simulink library "GRC_Lib"  (R2017b)
settings: Solver=VariableStepAuto  StartTime=0.0  StopTime=10.0  RelTol=1e-3  EnableMultiTasking=on
StartFcn:
  | set_param('AdvancedOperations','ZoomFactor','100');
undefined symbols (not defined in the file): Test
libraries: GRC_Lib x203, simulink x1
(part 4 of 4)

== system GRC_Lib/ComparationOperation/aub ==
  Max : Inport
      settings: AttributesFormatString=%<OutDataTypeStr>
  u : Inport  Port=2
      settings: AttributesFormatString=%<OutDataTypeStr>
  Min : Inport  Port=3
      settings: AttributesFormatString=%<OutDataTypeStr>
  Logical Operator : Logic  AllPortsSameDT=off  OutDataTypeStr=boolean
  Relational Operator : RelationalOperator  OutDataTypeStr=boolean  RndMeth=Nearest
  Relational Operator1 : RelationalOperator  OutDataTypeStr=boolean  RndMeth=Nearest
  y : Outport
      settings: AttributesFormatString=%<OutDataTypeStr>
  wires:
  Relational Operator/1 -> Logical Operator/1
  Relational Operator1/1 -> Logical Operator/2
  Logical Operator/1 -> y/1
  u/1 -> Relational Operator1/1, Relational Operator/2
  Max/1 -> Relational Operator/1
  Min/1 -> Relational Operator1/2

== system GRC_Lib/ComparationOperation/uab ==
  Max : Inport
      settings: AttributesFormatString=%<OutDataTypeStr>
  u : Inport  Port=2
      settings: AttributesFormatString=%<OutDataTypeStr>
  Min : Inport  Port=3
      settings: AttributesFormatString=%<OutDataTypeStr>
  Logical Operator : Logic  AllPortsSameDT=off  OutDataTypeStr=boolean
  Relational Operator : RelationalOperator  OutDataTypeStr=boolean  RndMeth=Nearest
  Relational Operator1 : RelationalOperator  Operator=>  OutDataTypeStr=boolean  RndMeth=Nearest
  y : Outport
      settings: AttributesFormatString=%<OutDataTypeStr>
  wires:
  Relational Operator/1 -> Logical Operator/1
  Relational Operator1/1 -> Logical Operator/2
  Logical Operator/1 -> y/1
  u/1 -> Relational Operator1/1, Relational Operator/2
  Max/1 -> Relational Operator/1
  Min/1 -> Relational Operator1/2

== system GRC_Lib/ComparationOperation/uabu ==
  Max : Inport
      settings: AttributesFormatString=%<OutDataTypeStr>
  u : Inport  Port=2
      settings: AttributesFormatString=%<OutDataTypeStr>
  Min : Inport  Port=3
      settings: AttributesFormatString=%<OutDataTypeStr>
  Logical Operator : Logic  AllPortsSameDT=off  OutDataTypeStr=boolean
  Relational Operator : RelationalOperator  Operator=>  OutDataTypeStr=boolean  RndMeth=Nearest
  Relational Operator1 : RelationalOperator  Operator=>  OutDataTypeStr=boolean  RndMeth=Nearest
  y : Outport
      settings: AttributesFormatString=%<OutDataTypeStr>
  wires:
  Relational Operator/1 -> Logical Operator/1
  Relational Operator1/1 -> Logical Operator/2
  Logical Operator/1 -> y/1
  u/1 -> Relational Operator1/1, Relational Operator/2
  Max/1 -> Relational Operator/1
  Min/1 -> Relational Operator1/2

== system GRC_Lib/Constants_Parameters/CalConstant ==
  CalParam : Constant  Value=CalParamName
  Out : Outport
  wires:
  CalParam/1 -> Out/1

== system GRC_Lib/Constants_Parameters/Stdrd1DLookupTable ==
  u : Inport
      settings: AttributesFormatString=%<OutDataTypeStr>
  Stdrd1DTable : Lookup_n-D  NumberOfTableDimensions=1  BreakpointsForDimension1=[-pi:pi/50:pi]  BreakpointsForDimension1DataTypeStr=double  Table=sin([-pi:pi/50:pi])  TableDataTypeStr=double  IntermediateResultsDataTypeStr=double  InternalRulePriority=Speed  OutDataTypeStr=double  RndMeth=Simplest  FractionDataTypeStr=double  InputSameDT=on
  y : Outport
      settings: AttributesFormatString=%<OutDataTypeStr>
  wires:
  u/1 -> Stdrd1DTable/1
  Stdrd1DTable/1 -> y/1

== system GRC_Lib/Constants_Parameters/Stdrd2DLookupTable ==
  x : Inport
      settings: AttributesFormatString=%<OutDataTypeStr>
  y : Inport  Port=2
      settings: AttributesFormatString=%<OutDataTypeStr>
  Stdrd2DTable : Lookup_n-D  BreakpointsForDimension1=[1 2 3 4]  BreakpointsForDimension2=[1 2 3]  BreakpointsForDimension1DataTypeStr=double  BreakpointsForDimension2DataTypeStr=double  Table=[4 5 6;15 17 19;10 15 23;5 13 20]  TableDataTypeStr=double  IntermediateResultsDataTypeStr=double  InternalRulePriority=Speed  OutDataTypeStr=double  RndMeth=Simplest  FractionDataTypeStr=double  InputSameDT=on
  out : Outport
      settings: AttributesFormatString=%<OutDataTypeStr>
  wires:
  x/1 -> Stdrd2DTable/1
  y/1 -> Stdrd2DTable/2
  Stdrd2DTable/1 -> out/1

== system GRC_Lib/Counter_Timer/RstCntDwn ==
  Rst : Inport
      settings: AttributesFormatString=%<OutDataTypeStr>
  RstV : Inport  Port=2
      settings: AttributesFormatString=%<OutDataTypeStr>
  E : Inport  Port=3
      settings: AttributesFormatString=%<OutDataTypeStr>
  AND : GRC_Lib/LogicalOperation/AND  n=2
  Big : GRC_Lib/ComparationOperation/Big  IpDT=double
  Big1 : GRC_Lib/ComparationOperation/Big  IpDT=double
  Constant : Constant  Value=0  OutDataTypeStr=uint16
      settings: AttributesFormatString=%<OutDataTypeStr>
  Constant1 : Constant  OutDataTypeStr=uint16
      settings: AttributesFormatString=%<OutDataTypeStr>
  Constant2 : Constant  Value=0  OutDataTypeStr=boolean
      settings: AttributesFormatString=%<OutDataTypeStr>
  Delay : GRC_Lib/Delay/Delay  IniV=1  IpDT=double
  SUB_Uint : GRC_Lib/ArithmeticOperations/SUB_Uint  IpDT=uint16
      settings: AttributesFormatString=SUB_Uint
  SWT3 : GRC_Lib/SignalSwitch/SWT3
  y : Outport
      settings: AttributesFormatString=%<OutDataTypeStr>
  wires:
  Rst/1 -> SWT3/1
  RstV/1 -> SWT3/2
  E/1 -> AND/1
  Big/1 -> AND/2
  Constant/1 -> Big/2
  SWT3/1 -> Big1/1, Delay/1
  Constant2/1 -> Big1/2
  Big1/1 -> y/1
  Constant1/1 -> SUB_Uint/2
  Delay/1 -> SUB_Uint/1, Big/1, SWT3/5
  SUB_Uint/1 -> SWT3/4
  AND/1 -> SWT3/3

== system GRC_Lib/Counter_Timer/RstCntStpRise ==
  Rst : Inport
      settings: AttributesFormatString=%<OutDataTypeStr>
  RstV : Inport  Port=2
      settings: AttributesFormatString=%<OutDataTypeStr>
  E : Inport  Port=3
      settings: AttributesFormatString=%<OutDataTypeStr>
  Constant : Constant  OutDataTypeStr=uint8
      settings: AttributesFormatString=%<OutDataTypeStr>
  DelayIniV : GRC_Lib/Delay/DelayIniV
  SUM : GRC_Lib/ArithmeticOperations/SUM  IpDT=uint8  OFChk=off
      settings: AttributesFormatString=%<IpDT>
  SWT3 : GRC_Lib/SignalSwitch/SWT3
  Cntr : Outport
      settings: AttributesFormatString=%<OutDataTypeStr>
  wires:
  Rst/1 -> SWT3/1
  RstV/1 -> SWT3/2, DelayIniV/1
  E/1 -> SWT3/3
  SWT3/1 -> Cntr/1, DelayIniV/2
  Constant/1 -> SUM/1
  DelayIniV/1 -> SWT3/5, SUM/2
  SUM/1 -> SWT3/4

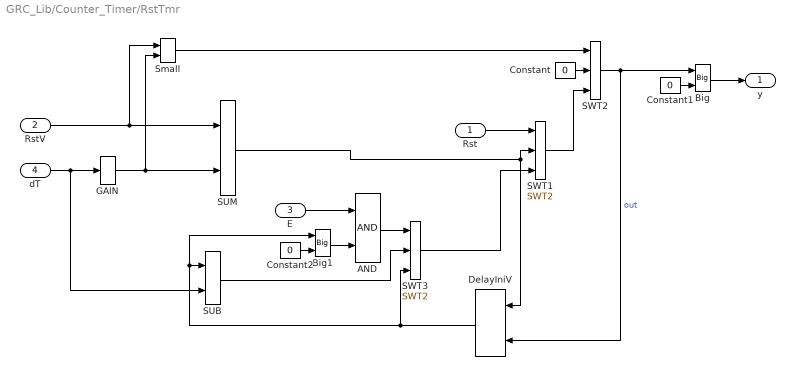
== system GRC_Lib/Counter_Timer/RstTmr ==
  Rst : Inport
      settings: AttributesFormatString=%<OutDataTypeStr>
  RstV : Inport  Port=2
      settings: AttributesFormatString=%<OutDataTypeStr>
  E : Inport  Port=3
      settings: AttributesFormatString=%<OutDataTypeStr>
  dT : Inport  Port=4
      settings: AttributesFormatString=%<OutDataTypeStr>
  AND : GRC_Lib/LogicalOperation/AND  n=2
  Big : GRC_Lib/ComparationOperation/Big  IpDT=double
  Big1 : GRC_Lib/ComparationOperation/Big  IpDT=double
  Constant : Constant  Value=0  OutDataTypeStr=double
      settings: AttributesFormatString=%<OutDataTypeStr>
  Constant1 : Constant  Value=0  OutDataTypeStr=double
      settings: AttributesFormatString=%<OutDataTypeStr>
  Constant2 : Constant  Value=0  OutDataTypeStr=double
      settings: AttributesFormatString=%<OutDataTypeStr>
  DelayIniV : GRC_Lib/Delay/DelayIniV
  GAIN : GRC_Lib/ArithmeticOperations/GAIN  K=0.5  IpDT=double  OFChk=on
      settings: AttributesFormatString=|
      | K=%<K>
      | %<IpDT>
  SUB : GRC_Lib/ArithmeticOperations/SUB  IpDT=double  OFChk=on
      settings: AttributesFormatString=%<IpDT>
  SUM : GRC_Lib/ArithmeticOperations/SUM  IpDT=double  OFChk=on
      settings: AttributesFormatString=%<IpDT>
  SWT1 : GRC_Lib/SignalSwitch/SWT2  OpDT=double
  SWT2 : GRC_Lib/SignalSwitch/SWT2  OpDT=double
  SWT3 : GRC_Lib/SignalSwitch/SWT2  OpDT=double
  Small : GRC_Lib/ComparationOperation/Small  IpDT=double
  y : Outport
      settings: AttributesFormatString=%<OutDataTypeStr>
  wires:
  dT/1 -> SUB/2, GAIN/1
  GAIN/1 -> SUM/2, Small/2
  RstV/1 -> SUM/1, Small/1
  E/1 -> AND/1
  Small/1 -> SWT2/1
  Constant/1 -> SWT2/2
  SWT2/1 -> DelayIniV/2, Big/1  "out"
  Constant1/1 -> Big/2
  Big/1 -> y/1
  SWT1/1 -> SWT2/3
  SUM/1 -> SWT1/2, DelayIniV/1
  SWT3/1 -> SWT1/3
  DelayIniV/1 -> SUB/1, Big1/1, SWT3/3
  SUB/1 -> SWT3/2
  Constant2/1 -> Big1/2
  Big1/1 -> AND/2
  AND/1 -> SWT3/1
  Rst/1 -> SWT1/1

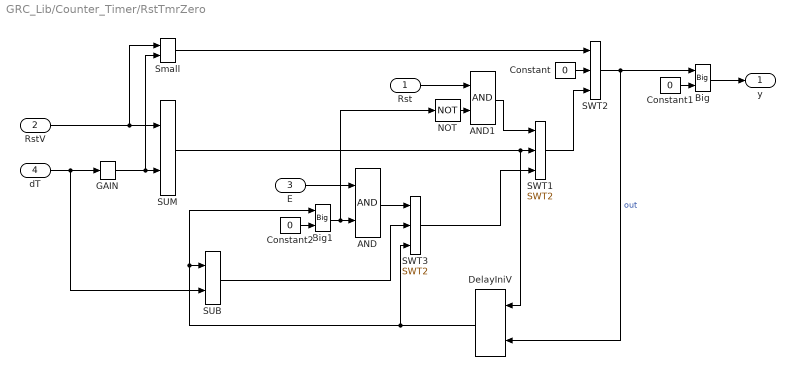
== system GRC_Lib/Counter_Timer/RstTmrZero ==
  Rst : Inport
      settings: AttributesFormatString=%<OutDataTypeStr>
  RstV : Inport  Port=2
      settings: AttributesFormatString=%<OutDataTypeStr>
  E : Inport  Port=3
      settings: AttributesFormatString=%<OutDataTypeStr>
  dT : Inport  Port=4
      settings: AttributesFormatString=%<OutDataTypeStr>
  AND : GRC_Lib/LogicalOperation/AND  n=2
  AND1 : GRC_Lib/LogicalOperation/AND  n=2
  Big : GRC_Lib/ComparationOperation/Big  IpDT=double
  Big1 : GRC_Lib/ComparationOperation/Big  IpDT=double
  Constant : Constant  Value=0  OutDataTypeStr=double
      settings: AttributesFormatString=%<OutDataTypeStr>
  Constant1 : Constant  Value=0  OutDataTypeStr=double
      settings: AttributesFormatString=%<OutDataTypeStr>
  Constant2 : Constant  Value=0  OutDataTypeStr=double
      settings: AttributesFormatString=%<OutDataTypeStr>
  DelayIniV : GRC_Lib/Delay/DelayIniV
  GAIN : GRC_Lib/ArithmeticOperations/GAIN  K=0.5  IpDT=double  OFChk=on
      settings: AttributesFormatString=|
      | K=%<K>
      | %<IpDT>
  NOT : GRC_Lib/LogicalOperation/NOT
  SUB : GRC_Lib/ArithmeticOperations/SUB  IpDT=double  OFChk=on
      settings: AttributesFormatString=%<IpDT>
  SUM : GRC_Lib/ArithmeticOperations/SUM  IpDT=double  OFChk=on
      settings: AttributesFormatString=%<IpDT>
  SWT1 : GRC_Lib/SignalSwitch/SWT2  OpDT=double
  SWT2 : GRC_Lib/SignalSwitch/SWT2  OpDT=double
  SWT3 : GRC_Lib/SignalSwitch/SWT2  OpDT=double
  Small : GRC_Lib/ComparationOperation/Small  IpDT=double
  y : Outport
      settings: AttributesFormatString=%<OutDataTypeStr>
  wires:
  dT/1 -> SUB/2, GAIN/1
  GAIN/1 -> Small/2, SUM/2
  RstV/1 -> Small/1, SUM/1
  E/1 -> AND/1
  Small/1 -> SWT2/1
  Constant/1 -> SWT2/2
  SWT2/1 -> DelayIniV/2, Big/1  "out"
  Constant1/1 -> Big/2
  Big/1 -> y/1
  SWT1/1 -> SWT2/3
  SUM/1 -> SWT1/2, DelayIniV/1
  SWT3/1 -> SWT1/3
  DelayIniV/1 -> Big1/1, SUB/1, SWT3/3
  SUB/1 -> SWT3/2
  Constant2/1 -> Big1/2
  Big1/1 -> NOT/1, AND/2
  AND/1 -> SWT3/1
  NOT/1 -> AND1/2
  Rst/1 -> AND1/1
  AND1/1 -> SWT1/1

== system GRC_Lib/Counter_Timer/StopWatch ==
  Rst : Inport
      settings: AttributesFormatString=%<OutDataTypeStr>
  E : Inport  Port=2
      settings: AttributesFormatString=%<OutDataTypeStr>
  dT : Inport  Port=3
      settings: AttributesFormatString=%<OutDataTypeStr>
  Constant : Constant  Value=0.0  OutDataTypeStr=single
      settings: AttributesFormatString=%<OutDataTypeStr>
  Delay : GRC_Lib/Delay/Delay  IniV=0  IpDT=double
  SUM : GRC_Lib/ArithmeticOperations/SUM  IpDT=single  OFChk=on
      settings: AttributesFormatString=%<IpDT>
  SWT3 : GRC_Lib/SignalSwitch/SWT3
  Tmr : Outport
      settings: AttributesFormatString=%<OutDataTypeStr>
  wires:
  Rst/1 -> SWT3/1
  E/1 -> SWT3/3
  Constant/1 -> SWT3/2
  SWT3/1 -> Delay/1, Tmr/1
  dT/1 -> SUM/1
  Delay/1 -> SWT3/5, SUM/2
  SUM/1 -> SWT3/4

== system GRC_Lib/Delay/Delay ==
  u : Inport
      settings: AttributesFormatString=%<OutDataTypeStr>
  UnitDelay : UnitDelay  SampleTime=-1
  y : Outport  InitialOutput=0
      settings: AttributesFormatString=%<OutDataTypeStr>
  wires:
  u/1 -> UnitDelay/1
  UnitDelay/1 -> y/1

== system GRC_Lib/Delay/DelayIniV ==
  IniV : Inport
      settings: AttributesFormatString=%<OutDataTypeStr>
  u : Inport  Port=2
      settings: AttributesFormatString=%<OutDataTypeStr>
  Constant : Constant  Value=0  OutDataTypeStr=boolean
  Delay : GRC_Lib/Delay/Delay  IniV=1  IpDT=double
  Delay1 : GRC_Lib/Delay/Delay  IniV=0  IpDT=double
  SWT2 : GRC_Lib/SignalSwitch/SWT2  OpDT=double
  y : Outport
      settings: AttributesFormatString=%<OutDataTypeStr>
  wires:
  Constant/1 -> Delay/1
  Delay/1 -> SWT2/1
  IniV/1 -> SWT2/2
  u/1 -> Delay1/1
  Delay1/1 -> SWT2/3
  SWT2/1 -> y/1

== system GRC_Lib/Delay/InitStp ==
  Cnst : Constant  Value=0  OutDataTypeStr=boolean
  Delay : UnitDelay  InitialCondition=1  SampleTime=-1
  y : Outport
      settings: AttributesFormatString=%<OutDataTypeStr>
  wires:
  Delay/1 -> y/1
  Cnst/1 -> Delay/1

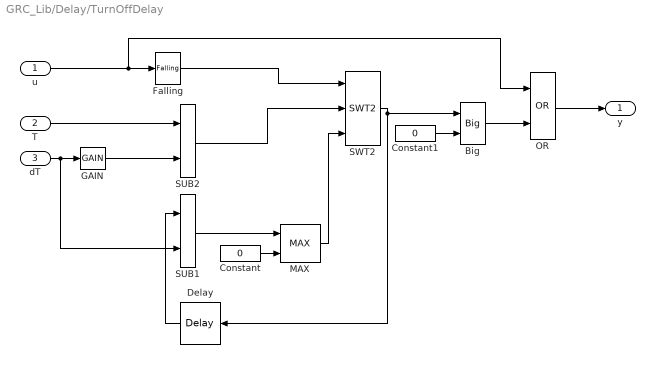
== system GRC_Lib/Delay/TurnOffDelay ==
  u : Inport
      settings: AttributesFormatString=%<OutDataTypeStr>
  T : Inport  Port=2
      settings: AttributesFormatString=%<OutDataTypeStr>
  dT : Inport  Port=3
      settings: AttributesFormatString=%<OutDataTypeStr>
  Big : GRC_Lib/ComparationOperation/Big  IpDT=double
  Constant : Constant  Value=0  OutDataTypeStr=double
  Constant1 : Constant  Value=0  OutDataTypeStr=double
  Delay : GRC_Lib/Delay/Delay  IniV=0  IpDT=double
  Falling : GRC_Lib/Memory/Falling  IniVal=0
  GAIN : GRC_Lib/ArithmeticOperations/GAIN  K=0.5  IpDT=double  OFChk=on
      settings: AttributesFormatString=|
      | K=%<K>
      | %<IpDT>
  MAX : GRC_Lib/ComparationOperation/MAX  OpDT=double
  OR : GRC_Lib/LogicalOperation/OR  n=2
  SUB1 : GRC_Lib/ArithmeticOperations/SUB  IpDT=double  OFChk=on
  SUB2 : GRC_Lib/ArithmeticOperations/SUB  IpDT=double  OFChk=on
  SWT2 : GRC_Lib/SignalSwitch/SWT2  OpDT=double
  y : Outport
      settings: AttributesFormatString=%<OutDataTypeStr>
  wires:
  u/1 -> OR/1, Falling/1
  Falling/1 -> SWT2/1
  T/1 -> SUB2/1
  GAIN/1 -> SUB2/2
  SUB2/1 -> SWT2/2
  dT/1 -> SUB1/2, GAIN/1
  Delay/1 -> SUB1/1
  SUB1/1 -> MAX/1
  Constant/1 -> MAX/2
  MAX/1 -> SWT2/3
  SWT2/1 -> Delay/1, Big/1
  Constant1/1 -> Big/2
  Big/1 -> OR/2
  OR/1 -> y/1

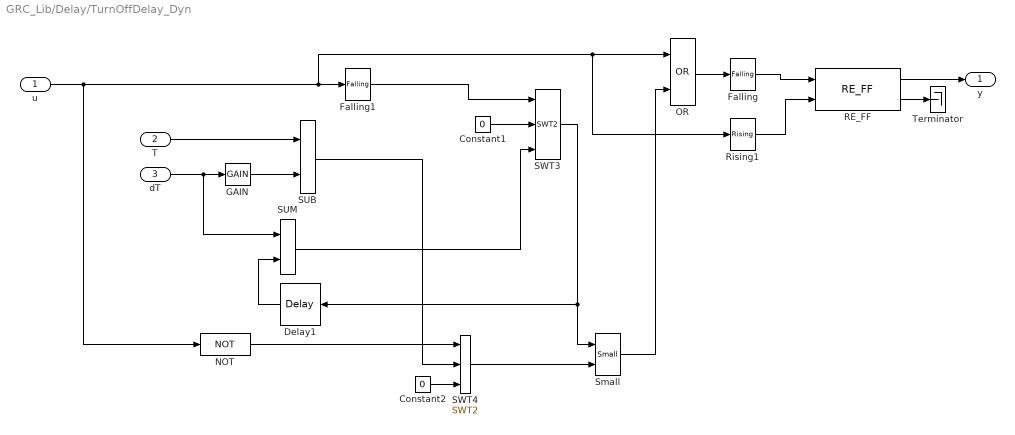
== system GRC_Lib/Delay/TurnOffDelay_Dyn ==
  u : Inport
      settings: AttributesFormatString=%<OutDataTypeStr>
  T : Inport  Port=2
      settings: AttributesFormatString=%<OutDataTypeStr>
  dT : Inport  Port=3
      settings: AttributesFormatString=%<OutDataTypeStr>
  Constant1 : Constant  Value=0  OutDataTypeStr=double
  Constant2 : Constant  Value=0  OutDataTypeStr=double
  Delay1 : GRC_Lib/Delay/Delay  IniV=0  IpDT=double
  Falling : GRC_Lib/Memory/Falling  IniVal=0
  Falling1 : GRC_Lib/Memory/Falling  IniVal=0
  GAIN : GRC_Lib/ArithmeticOperations/GAIN  K=0.5  IpDT=double  OFChk=on
      settings: AttributesFormatString=|
      | K=%<K>
      | %<IpDT>
  NOT : GRC_Lib/LogicalOperation/NOT
  OR : GRC_Lib/LogicalOperation/OR  n=2
  RE_FF : GRC_Lib/Memory/RE_FF  FalseVal=0  TrueVal=1
  Rising1 : GRC_Lib/Memory/Rising  IniVal=0
  SUB : GRC_Lib/ArithmeticOperations/SUB  IpDT=double  OFChk=on
  SUM : GRC_Lib/ArithmeticOperations/SUM  IpDT=double  OFChk=on
  SWT3 : GRC_Lib/SignalSwitch/SWT2  OpDT=double
  SWT4 : GRC_Lib/SignalSwitch/SWT2  OpDT=double
  Small : GRC_Lib/ComparationOperation/Small  IpDT=double
  Terminator : Terminator
  y : Outport
      settings: AttributesFormatString=%<OutDataTypeStr>
  wires:
  RE_FF/2 -> Terminator/1
  RE_FF/1 -> y/1
  Rising1/1 -> RE_FF/2
  Falling/1 -> RE_FF/1
  NOT/1 -> SWT4/1
  Small/1 -> OR/2
  SWT4/1 -> Small/2
  u/1 -> Falling1/1, OR/1, Rising1/1, NOT/1
  OR/1 -> Falling/1
  Constant1/1 -> SWT3/2
  Constant2/1 -> SWT4/3
  SWT3/1 -> Delay1/1, Small/1
  SUM/1 -> SWT3/3
  Delay1/1 -> SUM/2
  dT/1 -> GAIN/1, SUM/1
  SUB/1 -> SWT4/2
  GAIN/1 -> SUB/2
  T/1 -> SUB/1
  Falling1/1 -> SWT3/1

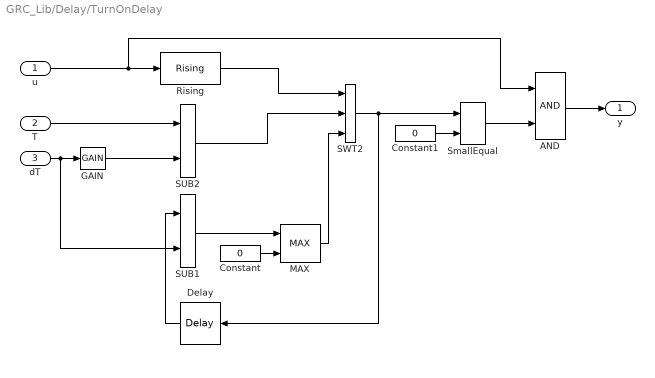
== system GRC_Lib/Delay/TurnOnDelay ==
  u : Inport
      settings: AttributesFormatString=%<OutDataTypeStr>
  T : Inport  Port=2
      settings: AttributesFormatString=%<OutDataTypeStr>
  dT : Inport  Port=3
      settings: AttributesFormatString=%<OutDataTypeStr>
  AND : GRC_Lib/LogicalOperation/AND  n=2
  Constant : Constant  Value=0  OutDataTypeStr=double
  Constant1 : Constant  Value=0  OutDataTypeStr=double
  Delay : GRC_Lib/Delay/Delay  IniV=0  IpDT=double
  GAIN : GRC_Lib/ArithmeticOperations/GAIN  K=0.5  IpDT=double  OFChk=on
      settings: AttributesFormatString=|
      | K=%<K>
      | %<IpDT>
  MAX : GRC_Lib/ComparationOperation/MAX  OpDT=double
  Rising : GRC_Lib/Memory/Rising  IniVal=0
  SUB1 : GRC_Lib/ArithmeticOperations/SUB  IpDT=double  OFChk=on
  SUB2 : GRC_Lib/ArithmeticOperations/SUB  IpDT=double  OFChk=on
  SWT2 : GRC_Lib/SignalSwitch/SWT2  OpDT=double
  SmallEqual : GRC_Lib/ComparationOperation/SmallEqual  IpDT=double
  y : Outport
      settings: AttributesFormatString=%<OutDataTypeStr>
  wires:
  u/1 -> AND/1, Rising/1
  Rising/1 -> SWT2/1
  T/1 -> SUB2/1
  GAIN/1 -> SUB2/2
  SUB2/1 -> SWT2/2
  dT/1 -> SUB1/2, GAIN/1
  Delay/1 -> SUB1/1
  SUB1/1 -> MAX/1
  Constant/1 -> MAX/2
  MAX/1 -> SWT2/3
  SWT2/1 -> SmallEqual/1, Delay/1
  Constant1/1 -> SmallEqual/2
  SmallEqual/1 -> AND/2
  AND/1 -> y/1

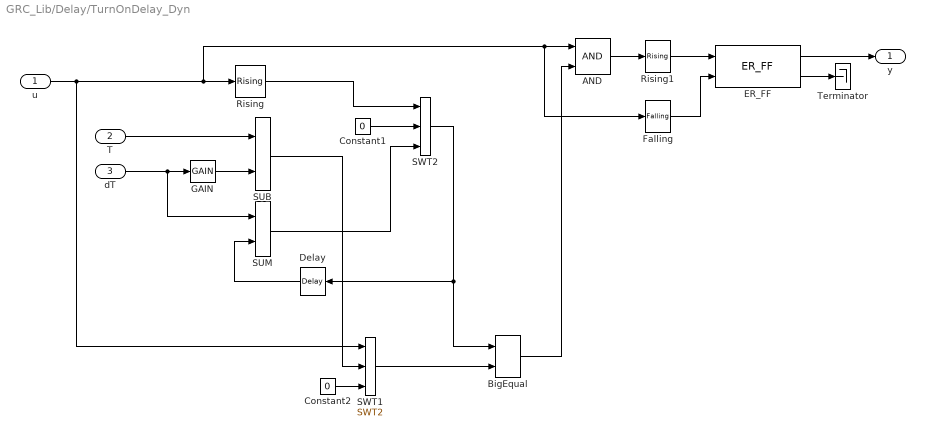
== system GRC_Lib/Delay/TurnOnDelay_Dyn ==
  u : Inport
      settings: AttributesFormatString=%<OutDataTypeStr>
  T : Inport  Port=2
      settings: AttributesFormatString=%<OutDataTypeStr>
  dT : Inport  Port=3
      settings: AttributesFormatString=%<OutDataTypeStr>
  AND : GRC_Lib/LogicalOperation/AND  n=2
  BigEqual : GRC_Lib/ComparationOperation/BigEqual  IpDT=double
  Constant1 : Constant  Value=0  OutDataTypeStr=single
  Constant2 : Constant  Value=0  OutDataTypeStr=single
  Delay : GRC_Lib/Delay/Delay  IniV=0  IpDT=double
  ER_FF : GRC_Lib/Memory/ER_FF  FalseVal=0  TrueVal=1
  Falling : GRC_Lib/Memory/Falling  IniVal=0
  GAIN : GRC_Lib/ArithmeticOperations/GAIN  K=0.5  IpDT=single  OFChk=on
      settings: AttributesFormatString=|
      | K=%<K>
      | %<IpDT>
  Rising : GRC_Lib/Memory/Rising  IniVal=0
  Rising1 : GRC_Lib/Memory/Rising  IniVal=0
  SUB : GRC_Lib/ArithmeticOperations/SUB  IpDT=single  OFChk=on
  SUM : GRC_Lib/ArithmeticOperations/SUM  IpDT=single  OFChk=on
  SWT1 : GRC_Lib/SignalSwitch/SWT2  OpDT=double
  SWT2 : GRC_Lib/SignalSwitch/SWT2  OpDT=double
  Terminator : Terminator
  y : Outport
      settings: AttributesFormatString=%<OutDataTypeStr>
  wires:
  ER_FF/2 -> Terminator/1
  Falling/1 -> ER_FF/2
  Rising1/1 -> ER_FF/1
  ER_FF/1 -> y/1
  AND/1 -> Rising1/1
  BigEqual/1 -> AND/2
  u/1 -> AND/1, Falling/1, Rising/1, SWT1/1
  Constant1/1 -> SWT2/2
  SWT1/1 -> BigEqual/2
  Constant2/1 -> SWT1/3
  Rising/1 -> SWT2/1
  GAIN/1 -> SUB/2
  SUB/1 -> SWT1/2
  dT/1 -> GAIN/1, SUM/1
  Delay/1 -> SUM/2
  SUM/1 -> SWT2/3
  T/1 -> SUB/1
  SWT2/1 -> Delay/1, BigEqual/1

== system GRC_Lib/Filter/DigitalLowPass ==
  note: // Note
      | Yn = a*(Xn-Yn-1) + Yn-1
  Rst : Inport
      settings: AttributesFormatString=%<OutDataTypeStr>
  RstV : Inport  Port=2
      settings: AttributesFormatString=%<OutDataTypeStr>
  E : Inport  Port=3
      settings: AttributesFormatString=%<OutDataTypeStr>
  u : Inport  Port=4
      settings: AttributesFormatString=%<OutDataTypeStr>
  m : Inport  Port=5
      settings: AttributesFormatString=%<OutDataTypeStr>
  DelayIniV : GRC_Lib/Delay/DelayIniV
  MUL : GRC_Lib/ArithmeticOperations/MUL  IpDT=single  OFChk=off
  SUB : GRC_Lib/ArithmeticOperations/SUB  IpDT=single  OFChk=off
  SUM : GRC_Lib/ArithmeticOperations/SUM  IpDT=single  OFChk=off
  SWT3 : GRC_Lib/SignalSwitch/SWT3
  y : Outport
      settings: AttributesFormatString=%<OutDataTypeStr>
  wires:
  Rst/1 -> SWT3/1
  RstV/1 -> DelayIniV/1, SWT3/2
  SWT3/1 -> DelayIniV/2, y/1
  E/1 -> SWT3/3
  u/1 -> SUB/1
  DelayIniV/1 -> SUM/2, SUB/2, SWT3/5
  SUB/1 -> MUL/2
  m/1 -> MUL/1
  MUL/1 -> SUM/1
  SUM/1 -> SWT3/4

== system GRC_Lib/Filter/LowPass_NoTrigger ==
  note: // Note,一阶低通滤波
      | Yn = a*(Xn-Yn-1) + Yn-1
  u : Inport
      settings: AttributesFormatString=%<OutDataTypeStr>
  m : Inport  Port=2
      settings: AttributesFormatString=%<OutDataTypeStr>
  Delay : GRC_Lib/Delay/Delay  IniV=0  IpDT=double
  MUL : GRC_Lib/ArithmeticOperations/MUL  IpDT=double  OFChk=off
  SUB : GRC_Lib/ArithmeticOperations/SUB  IpDT=double  OFChk=off
  SUM : GRC_Lib/ArithmeticOperations/SUM  IpDT=double  OFChk=off
  y : Outport
      settings: AttributesFormatString=%<OutDataTypeStr>
  wires:
  MUL/1 -> SUM/1
  m/1 -> MUL/1
  Delay/1 -> SUM/2, SUB/2
  SUB/1 -> MUL/2
  SUM/1 -> y/1, Delay/1
  u/1 -> SUB/1

== system GRC_Lib/Intergrator/Accumulator ==
  Max : Inport
      settings: AttributesFormatString=%<OutDataTypeStr>
  Min : Inport  Port=2
      settings: AttributesFormatString=%<OutDataTypeStr>
  Rst : Inport  Port=3
      settings: AttributesFormatString=%<OutDataTypeStr>
  RstV : Inport  Port=4
      settings: AttributesFormatString=%<OutDataTypeStr>
  E : Inport  Port=5
      settings: AttributesFormatString=%<OutDataTypeStr>
  u : Inport  Port=6
      settings: AttributesFormatString=%<OutDataTypeStr>
  Delay : GRC_Lib/Delay/Delay  IniV=0  IpDT=double
  LIMIT : GRC_Lib/Nonlinear/LIMIT  IpDT=double
  SUM : GRC_Lib/ArithmeticOperations/SUM  IpDT=int16  OFChk=off
  SWT3 : GRC_Lib/SignalSwitch/SWT3
  y : Outport
      settings: AttributesFormatString=%<OutDataTypeStr>
  MX_Flg : Outport  Port=2
      settings: AttributesFormatString=%<OutDataTypeStr>
  MN_Flg : Outport  Port=3
      settings: AttributesFormatString=%<OutDataTypeStr>
  wires:
  Delay/1 -> SUM/2, SWT3/5
  LIMIT/1 -> Delay/1, y/1
  LIMIT/2 -> MX_Flg/1
  LIMIT/3 -> MN_Flg/1
  Min/1 -> LIMIT/3
  Max/1 -> LIMIT/1
  SWT3/1 -> LIMIT/2
  Rst/1 -> SWT3/1
  RstV/1 -> SWT3/2
  E/1 -> SWT3/3
  u/1 -> SUM/1
  SUM/1 -> SWT3/4

== system GRC_Lib/LogicalOperation/AND ==
  In1 : Inport
      settings: AttributesFormatString=%<OutDataTypeStr>
  In2 : Inport  Port=2
      settings: AttributesFormatString=%<OutDataTypeStr>
  AND1 : Logic  AllPortsSameDT=off  OutDataTypeStr=boolean
  Out : Outport
      settings: AttributesFormatString=%<OutDataTypeStr>
  wires:
  AND1/1 -> Out/1
  In1/1 -> AND1/1
  In2/1 -> AND1/2

== system GRC_Lib/LogicalOperation/NOT ==
  In1 : Inport
      settings: AttributesFormatString=%<OutDataTypeStr>
  NOT1 : Logic  Operator=NOT  Inputs=n  OutDataTypeStr=boolean
  Out : Outport
      settings: AttributesFormatString=%<OutDataTypeStr>
  wires:
  In1/1 -> NOT1/1
  NOT1/1 -> Out/1

== system GRC_Lib/LogicalOperation/OR ==
  In1 : Inport
      settings: AttributesFormatString=%<OutDataTypeStr>
  In2 : Inport  Port=2
      settings: AttributesFormatString=%<OutDataTypeStr>
  OR1 : Logic  Operator=OR  AllPortsSameDT=off  OutDataTypeStr=boolean
  Out : Outport
      settings: AttributesFormatString=%<OutDataTypeStr>
  wires:
  In2/1 -> OR1/2
  In1/1 -> OR1/1
  OR1/1 -> Out/1

== system GRC_Lib/LogicalOperation/XOR ==
  In1 : Inport
      settings: AttributesFormatString=%<OutDataTypeStr>
  In2 : Inport  Port=2
      settings: AttributesFormatString=%<OutDataTypeStr>
  XOR1 : Logic  Operator=XOR  AllPortsSameDT=off  OutDataTypeStr=boolean
  Out : Outport
      settings: AttributesFormatString=%<OutDataTypeStr>
  wires:
  XOR1/1 -> Out/1
  In1/1 -> XOR1/1
  In2/1 -> XOR1/2

== system GRC_Lib/MathFunction/Sqr ==
  u : Inport
      settings: AttributesFormatString=%<OutDataTypeStr>
  Square : Math  Operator=square  OutDataTypeStr=uint32  SaturateOnIntegerOverflow=on
      settings: AttributesFormatString=%<OutDataTypeStr>
  y : Outport
      settings: AttributesFormatString=%<OutDataTypeStr>
  wires:
  Square/1 -> y/1
  u/1 -> Square/1

== system GRC_Lib/MathFunction/Sqrt ==
  u : Inport
      settings: AttributesFormatString=%<OutDataTypeStr>
  Sqrt : Sqrt  OutDataTypeStr=double  SaturateOnIntegerOverflow=on
      settings: AttributesFormatString=%<OutDataTypeStr>
  y : Outport
      settings: AttributesFormatString=%<OutDataTypeStr>
  wires:
  Sqrt/1 -> y/1
  u/1 -> Sqrt/1

== system GRC_Lib/Memory/ER_FF ==
  E1_T : Inport
      settings: AttributesFormatString=%<OutDataTypeStr>
  R2_F : Inport  Port=2
      settings: AttributesFormatString=%<OutDataTypeStr>
  Delay : GRC_Lib/Delay/Delay  IniV=0  IpDT=double
  NOT : GRC_Lib/LogicalOperation/NOT
  SWT1 : GRC_Lib/SignalSwitch/SWT2  OpDT=double
  SWT2 : GRC_Lib/SignalSwitch/SWT2  OpDT=double
  false : Constant  Value=falseVal  OutDataTypeStr=boolean
  true : Constant  Value=trueVal  OutDataTypeStr=boolean
  y : Outport
      settings: AttributesFormatString=%<OutDataTypeStr>
  ~y : Outport  Port=2
      settings: AttributesFormatString=%<OutDataTypeStr>
  wires:
  E1_T/1 -> SWT2/1
  true/1 -> SWT2/2
  SWT1/1 -> SWT2/3
  R2_F/1 -> SWT1/1
  false/1 -> SWT1/2
  Delay/1 -> SWT1/3
  SWT2/1 -> Delay/1, NOT/1, y/1
  NOT/1 -> ~y/1

== system GRC_Lib/Memory/Falling ==
  In1 : Inport
      settings: AttributesFormatString=%<OutDataTypeStr>
  AND : GRC_Lib/LogicalOperation/AND  n=2
  Delay : GRC_Lib/Delay/Delay  IniV=0  IpDT=double
  NOT : GRC_Lib/LogicalOperation/NOT
  Out1 : Outport
      settings: AttributesFormatString=%<OutDataTypeStr>
  wires:
  AND/1 -> Out1/1
  Delay/1 -> AND/2
  NOT/1 -> AND/1
  In1/1 -> NOT/1, Delay/1

== system GRC_Lib/Memory/RE_FF ==
  R1_F : Inport
      settings: AttributesFormatString=%<OutDataTypeStr>
  E2_T : Inport  Port=2
      settings: AttributesFormatString=%<OutDataTypeStr>
  Delay : GRC_Lib/Delay/Delay  IniV=0  IpDT=double
  NOT : GRC_Lib/LogicalOperation/NOT
  SWT1 : GRC_Lib/SignalSwitch/SWT2  OpDT=double
  SWT2 : GRC_Lib/SignalSwitch/SWT2  OpDT=double
  false : Constant  Value=falseVal  OutDataTypeStr=boolean
  true : Constant  Value=trueVal  OutDataTypeStr=boolean
  y : Outport
      settings: AttributesFormatString=%<OutDataTypeStr>
  ~y : Outport  Port=2
      settings: AttributesFormatString=%<OutDataTypeStr>
  wires:
  NOT/1 -> ~y/1
  SWT1/1 -> y/1, NOT/1, Delay/1
  Delay/1 -> SWT2/3
  true/1 -> SWT2/2
  E2_T/1 -> SWT2/1
  SWT2/1 -> SWT1/3
  false/1 -> SWT1/2
  R1_F/1 -> SWT1/1

== system GRC_Lib/Memory/Rising ==
  In1 : Inport
      settings: AttributesFormatString=%<OutDataTypeStr>
  AND : GRC_Lib/LogicalOperation/AND  n=2
  Delay : GRC_Lib/Delay/Delay  IniV=0  IpDT=double
  NOT : GRC_Lib/LogicalOperation/NOT
  Out1 : Outport
      settings: AttributesFormatString=%<OutDataTypeStr>
  wires:
  NOT/1 -> AND/2
  Delay/1 -> NOT/1
  AND/1 -> Out1/1
  In1/1 -> Delay/1, AND/1

== system GRC_Lib/Memory/RisingFaling ==
  In1 : Inport
      settings: AttributesFormatString=%<OutDataTypeStr>
  Delay : GRC_Lib/Delay/Delay  IniV=0  IpDT=double
  XOR : GRC_Lib/LogicalOperation/XOR  n=2
  Out1 : Outport
      settings: AttributesFormatString=%<OutDataTypeStr>
  wires:
  Delay/1 -> XOR/2
  XOR/1 -> Out1/1
  In1/1 -> Delay/1, XOR/1

== system GRC_Lib/Nonlinear/ABS ==
  u : Inport
      settings: AttributesFormatString=%<OutDataTypeStr>
  Big : GRC_Lib/ComparationOperation/Big  IpDT=double
  Constant : Constant  Value=-1  OutDataTypeStr=int16
  Constant1 : Constant  Value=0  OutDataTypeStr=int16
  Product : Product  OutDataTypeStr=int16  SaturateOnIntegerOverflow=on  RndMeth=Zero
  SWT2 : GRC_Lib/SignalSwitch/SWT2  OpDT=double
  y : Outport
      settings: AttributesFormatString=%<OutDataTypeStr>
  wires:
  Constant/1 -> Product/2
  u/1 -> Big/1, SWT2/2, Product/1
  Constant1/1 -> Big/2
  Big/1 -> SWT2/1
  Product/1 -> SWT2/3
  SWT2/1 -> y/1

== system GRC_Lib/Nonlinear/HysLDlt ==
  D : Inport
      settings: AttributesFormatString=%<OutDataTypeStr>
  L : Inport  Port=2
      settings: AttributesFormatString=%<OutDataTypeStr>
  u : Inport  Port=3
      settings: AttributesFormatString=%<OutDataTypeStr>
  Big : GRC_Lib/ComparationOperation/Big  IpDT=double
  Delay : GRC_Lib/Delay/Delay  IniV=0  IpDT=double
  OR : GRC_Lib/LogicalOperation/OR  n=2
  SUM : GRC_Lib/ArithmeticOperations/SUM  IpDT=single  OFChk=on
  SWT2 : GRC_Lib/SignalSwitch/SWT2  OpDT=double
  Small : GRC_Lib/ComparationOperation/Small  IpDT=double
  y : Outport
      settings: AttributesFormatString=%<OutDataTypeStr>
  wires:
  SWT2/1 -> Delay/1, y/1
  u/1 -> Big/1, Small/1
  L/1 -> Small/2, SUM/1
  SUM/1 -> Big/2
  D/1 -> SUM/2
  Small/1 -> OR/1
  Big/1 -> SWT2/2, OR/2
  OR/1 -> SWT2/1
  Delay/1 -> SWT2/3

== system GRC_Lib/Nonlinear/HysRDlt ==
  R : Inport
      settings: AttributesFormatString=%<OutDataTypeStr>
  D : Inport  Port=2
      settings: AttributesFormatString=%<OutDataTypeStr>
  u : Inport  Port=3
      settings: AttributesFormatString=%<OutDataTypeStr>
  Big : GRC_Lib/ComparationOperation/Big  IpDT=double
  Delay : GRC_Lib/Delay/Delay  IniV=0  IpDT=double
  OR : GRC_Lib/LogicalOperation/OR  n=2
  SUB : GRC_Lib/ArithmeticOperations/SUB  IpDT=double  OFChk=on
  SWT2 : GRC_Lib/SignalSwitch/SWT2  OpDT=double
  Small : GRC_Lib/ComparationOperation/Small  IpDT=double
  y : Outport
      settings: AttributesFormatString=%<OutDataTypeStr>
  wires:
  D/1 -> SUB/2
  R/1 -> SUB/1, Big/2
  u/1 -> Small/1, Big/1
  SUB/1 -> Small/2
  Small/1 -> OR/1
  Big/1 -> SWT2/2, OR/2
  OR/1 -> SWT2/1
  SWT2/1 -> Delay/1, y/1
  Delay/1 -> SWT2/3

== system GRC_Lib/Nonlinear/Hysterisis ==
  Rst : Inport
      settings: AttributesFormatString=%<OutDataTypeStr>
  RstV : Inport  Port=2
      settings: AttributesFormatString=%<OutDataTypeStr>
  LV : Inport  Port=3
      settings: AttributesFormatString=%<OutDataTypeStr>
  RV : Inport  Port=4
      settings: AttributesFormatString=%<OutDataTypeStr>
  u : Inport  Port=5
      settings: AttributesFormatString=%<OutDataTypeStr>
  Big : GRC_Lib/ComparationOperation/Big  IpDT=double
  Delay : GRC_Lib/Delay/Delay  IniV=0  IpDT=double
  OR : GRC_Lib/LogicalOperation/OR  n=2
  SWT1 : GRC_Lib/SignalSwitch/SWT2  OpDT=double
  SWT2 : GRC_Lib/SignalSwitch/SWT2  OpDT=double
  Small : GRC_Lib/ComparationOperation/Small  IpDT=double
  y : Outport
      settings: AttributesFormatString=%<OutDataTypeStr>
  wires:
  u/1 -> Small/1, Big/1
  LV/1 -> Small/2
  RV/1 -> Big/2
  Rst/1 -> SWT2/1
  RstV/1 -> SWT2/2
  Small/1 -> OR/1
  Big/1 -> SWT1/2, OR/2
  OR/1 -> SWT1/1
  Delay/1 -> SWT1/3
  SWT1/1 -> SWT2/3
  SWT2/1 -> Delay/1, y/1

== system GRC_Lib/Nonlinear/Hysterisis_NoRst ==
  LV : Inport
      settings: AttributesFormatString=%<OutDataTypeStr>
  RV : Inport  Port=2
      settings: AttributesFormatString=%<OutDataTypeStr>
  u : Inport  Port=3
      settings: AttributesFormatString=%<OutDataTypeStr>
  Big : GRC_Lib/ComparationOperation/Big  IpDT=double
  Delay : GRC_Lib/Delay/Delay  IniV=0  IpDT=double
  OR : GRC_Lib/LogicalOperation/OR  n=2
  SWT1 : GRC_Lib/SignalSwitch/SWT2  OpDT=double
  Small : GRC_Lib/ComparationOperation/Small  IpDT=double
  y : Outport
      settings: AttributesFormatString=%<OutDataTypeStr>
  wires:
  SWT1/1 -> Delay/1, y/1
  Delay/1 -> SWT1/3
  OR/1 -> SWT1/1
  Big/1 -> OR/2, SWT1/2
  Small/1 -> OR/1
  RV/1 -> Big/2
  LV/1 -> Small/2
  u/1 -> Big/1, Small/1

== system GRC_Lib/Nonlinear/LIMIT ==
  MX : Inport
      settings: AttributesFormatString=%<OutDataTypeStr>
  u : Inport  Port=2
      settings: AttributesFormatString=%<OutDataTypeStr>
  MN : Inport  Port=3
      settings: AttributesFormatString=%<OutDataTypeStr>
  AND : GRC_Lib/LogicalOperation/AND  n=2
  Big : GRC_Lib/ComparationOperation/Big  IpDT=double
  MAX : GRC_Lib/ComparationOperation/MAX  OpDT=int32
  MIN : GRC_Lib/ComparationOperation/MIN  OpDT=double
  NOT : GRC_Lib/LogicalOperation/NOT
  Small : GRC_Lib/ComparationOperation/Small  IpDT=double
  y : Outport
      settings: AttributesFormatString=%<OutDataTypeStr>
  MX_F : Outport  Port=2
      settings: AttributesFormatString=%<OutDataTypeStr>
  MN_F : Outport  Port=3
      settings: AttributesFormatString=%<OutDataTypeStr>
  wires:
  MX/1 -> Big/2, MIN/1
  u/1 -> Small/1, Big/1, MAX/1
  MN/1 -> Small/2, MAX/2
  Big/1 -> NOT/1, MX_F/1
  Small/1 -> AND/2
  NOT/1 -> AND/1
  AND/1 -> MN_F/1
  MAX/1 -> MIN/2
  MIN/1 -> y/1

== system GRC_Lib/Nonlinear/SIGN ==
  u : Inport
      settings: AttributesFormatString=%<OutDataTypeStr>
  Sign : Signum
  y : Outport
      settings: AttributesFormatString=%<OutDataTypeStr>
  wires:
  Sign/1 -> y/1
  u/1 -> Sign/1

== system GRC_Lib/Routing/Selector ==
  U : Inport
      settings: AttributesFormatString=%<OutDataTypeStr>
  Idx1_0 : Inport  Port=2
      settings: AttributesFormatString=%<OutDataTypeStr>
  Constant : Constant  Value=5  OutDataTypeStr=uint8
      settings: AttributesFormatString=%<OutDataTypeStr>
  MIN : GRC_Lib/ComparationOperation/MIN  OpDT=double
  Selector1 : Selector  IndexMode=Zero-based  InputPortWidth=SizeU  IndexOptions=Index vector (port)  Indices=[1 3]  OutputSizes=1
      settings: AttributesFormatString=%<InputPortWidth>
  Y : Outport
      settings: AttributesFormatString=%<OutDataTypeStr>
  wires:
  Idx1_0/1 -> MIN/1
  Constant/1 -> MIN/2
  MIN/1 -> Selector1/2
  Selector1/1 -> Y/1
  U/1 -> Selector1/1

== system GRC_Lib/Routing/Vbi_OilTempSensor ==
  In1 : Inport  OutMin=0  OutMax=100
  Out1 : Outport
  wires:
  In1/1 -> Out1/1  "Vbi_OilTempSensor"

== system GRC_Lib/SignalAttributes/DTC ==
  Idt : Inport
      settings: AttributesFormatString=%<OutDataTypeStr>
  DTC : DataTypeConversion  OutDataTypeStr=double
  Odt : Outport
      settings: AttributesFormatString=%<OutDataTypeStr>
  wires:
  Idt/1 -> DTC/1
  DTC/1 -> Odt/1

== system GRC_Lib/SignalSwitch/SWT2 ==
  S : Inport
      settings: AttributesFormatString=%<OutDataTypeStr>
  T : Inport  Port=2
      settings: AttributesFormatString=%<OutDataTypeStr>
  F : Inport  Port=3
      settings: AttributesFormatString=%<OutDataTypeStr>
  SWT : Switch  Criteria=u2 ~= 0
  y : Outport
      settings: AttributesFormatString=%<OutDataTypeStr>
  wires:
  T/1 -> SWT/1
  S/1 -> SWT/2
  F/1 -> SWT/3
  SWT/1 -> y/1

== system GRC_Lib/SignalSwitch/SWT3 ==
  R : Inport
      settings: AttributesFormatString=%<OutDataTypeStr>
  Rv : Inport  Port=2
      settings: AttributesFormatString=%<OutDataTypeStr>
  E : Inport  Port=3
      settings: AttributesFormatString=%<OutDataTypeStr>
  u : Inport  Port=4
      settings: AttributesFormatString=%<OutDataTypeStr>
  df : Inport  Port=5
      settings: AttributesFormatString=%<OutDataTypeStr>
  SWT1 : GRC_Lib/SignalSwitch/SWT2  OpDT=double
  SWT2 : GRC_Lib/SignalSwitch/SWT2  OpDT=double
  y : Outport
      settings: AttributesFormatString=%<OutDataTypeStr>
  wires:
  R/1 -> SWT1/1
  Rv/1 -> SWT1/2
  E/1 -> SWT2/1
  u/1 -> SWT2/2
  df/1 -> SWT2/3
  SWT2/1 -> SWT1/3
  SWT1/1 -> y/1

== system GRC_Lib/SignalSwitch/SWTM ==
  S : Inport
      settings: AttributesFormatString=%<OutDataTypeStr>
  C1 : Inport  Port=2
      settings: AttributesFormatString=%<OutDataTypeStr>
  C2 : Inport  Port=3
      settings: AttributesFormatString=%<OutDataTypeStr>
  dft : Inport  Port=4
  SWT : MultiPortSwitch  DataPortOrder=Zero-based contiguous  Inputs=2  DataPortIndices={1,2,[3,4,5],6,7,[8,9,10],[11,12,13],14,15}  DataPortForDefault=Additional data port  OutDataTypeStr=double
      settings: AttributesFormatString=%<OutDataTypeStr>
  y : Outport
      settings: AttributesFormatString=%<OutDataTypeStr>
  wires:
  SWT/1 -> y/1
  S/1 -> SWT/1
  C1/1 -> SWT/2
  C2/1 -> SWT/3
  dft/1 -> SWT/4

== stateflow chart GRC_Lib/BitOperations/BitOR/Chart ==
  (default) -> (junction 1)
  (junction 1) -> (junction 3) : {Out = In1 | In2;}
  data: In1 input; In2 input; Out output

== stateflow chart GRC_Lib/BitOperations/BitXOR/Chart ==
  (default) -> (junction 1)
  (junction 1) -> (junction 3) : {Out = In1^In2;}
  data: In1 input; In2 input; Out output

== stateflow chart GRC_Lib/BitOperations/BitAND/Chart ==
  (default) -> (junction 2)
  (junction 2) -> (junction 1) : {Out = In1 & In2;}
  data: In1 input; In2 input; Out output

== stateflow chart GRC_Lib/BitOperations/NOT/Chart ==
  (default) -> (junction 3)
  (junction 3) -> (junction 4) : {Out = ~In;}
      | % Out = rem((In+1),2);
  data: In input; Out output

== stateflow chart GRC_Lib/BitOperations/ClearBit_32bit/Chart ==
  state clearBit_32/
    clearBit_32 -> (junction 4)
    (junction 4) -> (junction 11) [order 1] : [position < data_length]
    (junction 11) -> (junction 1) [order 1] : [position == (data_length-1)]
    (junction 4) -> (junction 16) [order 2] : {Out = bitArray;}
    (junction 11) -> (junction 10) [order 2] : {Out = (bitArray & ~(one << position));}
    (junction 1) -> (junction 9) : {Out = (bitArray & msb_clear_flag);}
    (junction 10) -> (junction 16)
    (junction 9) -> (junction 10)
    (junction 16) -> clearBit_32
  (default) -> (junction 4)
  data: bitArray input; position input uint8; one input; msb_clear_flag input; data_length input uint8; Out output

== stateflow chart GRC_Lib/BitOperations/GetBit_32bit/Chart ==
  (default) -> (junction 2)
  (junction 2) -> (junction 3) [order 1] : [BitPos < data_length]
  (junction 2) -> (junction 11) [order 2] : {BitValue = 0;}
  (junction 3) -> (junction 1) : {BitValue = (Value>>BitPos)&1;}
  (junction 1) -> (junction 11)
  (junction 11) -> (junction 5)
  data: Value input; BitPos input; data_length input; BitValue output

== stateflow chart GRC_Lib/BitOperations/SetBit_32bit/Chart ==
  (default) -> (junction 3)
  (junction 3) -> (junction 13) [order 1] : [Enable && BitPos < data_length]
  (junction 13) -> (junction 2) [order 1] : [BitPos == (data_length -1)]
  (junction 3) -> (junction 11) [order 2] : {y=u;}
  (junction 13) -> (junction 8) [order 2] : {y=u|(1<<BitPos);}
  (junction 2) -> (junction 1) : {y = u|msb_set_flag;}
  (junction 8) -> (junction 11)
  (junction 1) -> (junction 8)
  (junction 11) -> (junction 6)
  data: Enable input; u input; BitPos input; data_length input; msb_set_flag input; y output

== stateflow chart GRC_Lib/BitOperations/AndBit_32bit/Chart ==
  (default) -> (junction 2)
  (junction 2) -> (junction 1) : {Out = !((In1 & In2)==0);}
  data: In1 input; In2 input; Out output

== stateflow chart GRC_Lib/BitOperations/SetBit_Count/Chart ==
  (default) -> (junction 1) : {
      | count = 0;
      | input = u;
      | }
  (junction 1) -> (junction 7) [order 1] : [input > 0]
  (junction 5) -> (junction 1)
  (junction 1) -> (junction 4) [order 2]
  (junction 7) -> (junction 5) : {
      | input &= (input- 1);
      | count += 1;
      | }
  data: u input; input local uint32; count output uint8

== stateflow chart GRC_Lib/BitOperations/BitClear_Filter/Chart ==
  state BitClear
    BitClear -> BitClear : {Out = In & ~Fltr;}
  (default) -> BitClear
  data: In input; Fltr input; Out output

== stateflow chart GRC_Lib/BitOperations/MSB/Chart ==
  (default) -> (junction 10) : {
      | Pos = 0;
      | idx = i;
      | input = u;
      | }
  (junction 10) -> (junction 12) [order 1] : [idx >= 0]
  (junction 12) -> (junction 8) [order 1] : [input & RefBin[idx]]
  (junction 3) -> (junction 10) : { idx =idx-1;}
  (junction 10) -> (junction 7) [order 2]
  (junction 12) -> (junction 3) [order 2]
  (junction 8) -> (junction 11) : {
      | Pos |= RefPos[idx];
      | input = input>>RefPos[idx];
      | }
  (junction 11) -> (junction 3)
  data: u input; i input; RefBin input size=5; RefPos input size=5; Pos output uint8; input local uint32; idx local int8

== stateflow chart GRC_Lib/AdvancedOperations/1D_LookupTableContrafunctional/Chart ==
  (default) -> (junction 9) : {len=0;
      | x=0;
      | err=1;}
  (junction 9) -> (junction 12) [order 2]
  (junction 9) -> (junction 1) [order 1] : [(sizeof(arrX)==sizeof(arrY) ) && (sizeof(arrX)/sizeof(arrX[0])>=2)]
      | {len=sizeof(arrX)/sizeof(arrX[0])}
  (junction 12) -> (junction 25)
  (junction 1) -> (junction 14) [order 2]
  (junction 14) -> (junction 25) [order 2]
  (junction 1) -> (junction 3) [order 1] : [arrX[len-1]>arrX[0]]
      | {i=0}
  (junction 14) -> (junction 32) [order 1] : [arrX[len-1]<arrX[0]]
      | {i=0}
  (junction 3) -> (junction 20) [order 2]
  (junction 20) -> (junction 27)
  (junction 27) -> (junction 25)
  (junction 32) -> (junction 27) [order 2]
  (junction 122) -> (junction 20)
  (junction 125) -> (junction 27)
  (junction 25) -> (junction 56)
  (junction 7) -> (junction 3) [order 2] : [i<len-1]
  (junction 24) -> (junction 32) [order 2] : [i<len-1]
  (junction 3) -> (junction 7) [order 1] : [arrX[i+1]>=arrX[i]]
      | {i=i+1;}
  (junction 32) -> (junction 24) [order 1] : [arrX[i+1]<=arrX[i]]
      | {i=i+1;}
  (junction 7) -> (junction 122) [order 3]
  (junction 24) -> (junction 125) [order 3]
  (junction 7) -> (junction 18) [order 1] : [i==len-1]
      | {xInc=1}
  (junction 24) -> (junction 28) [order 1] : [i==len]
      | {xInc=0}
  (junction 28) -> (junction 18)
  (junction 18) -> (junction 65) : {i=0}
  (junction 65) -> (junction 45) [order 2]
  (junction 45) -> (junction 56) [order 2]
  (junction 65) -> (junction 66) [order 1] : [arrY[len-1]>arrY[0]]
      | {i=1}
  (junction 45) -> (junction 57) [order 1] : [arrY[len-1]<arrY[0]]
      | {i=1}
  (junction 66) -> (junction 46) [order 2]
  (junction 46) -> (junction 58)
  (junction 58) -> (junction 56)
  (junction 56) -> (junction 117)
  (junction 57) -> (junction 58) [order 2]
  (junction 81) -> (junction 46)
  (junction 84) -> (junction 58)
  (junction 117) -> (junction 118) : {err=0}
  (junction 42) -> (junction 66) [order 2] : [i<len-1]
  (junction 52) -> (junction 57) [order 2] : [i<len-1]
  (junction 66) -> (junction 42) [order 1] : [arrY[i+1]>=arrY[i]]
      | {i=i+1;}
  (junction 57) -> (junction 52) [order 1] : [arrY[i+1]<=arrY[i]]
      | {i=i+1;}
  (junction 42) -> (junction 81) [order 3]
  (junction 52) -> (junction 84) [order 3]
  (junction 42) -> (junction 48) [order 1] : [i==len-1]
      | {yInc=1}
  (junction 52) -> (junction 55) [order 1] : [i==len-1]
      | {yInc=0}
  (junction 55) -> (junction 97) : {i=len-1}
  (junction 48) -> (junction 70) : {i=len-1}
  (junction 70) -> (junction 68) [order 1] : [y>=arrY[len-1]]
  (junction 68) -> (junction 69) : {x=arrX[len-1]}
  (junction 97) -> (junction 96) [order 1] : [y<=arrY[len-1]]
  (junction 96) -> (junction 95) : {x=arrX[len-1]}
  (junction 70) -> (junction 87) [order 2]
  (junction 69) -> (junction 79)
  (junction 97) -> (junction 93) [order 2]
  (junction 95) -> (junction 104)
  (junction 73) -> (junction 87) [order 2] : [i>=1]
  (junction 100) -> (junction 93) [order 2] : [i>=1]
  (junction 87) -> (junction 73) : {i=i-1}
  (junction 93) -> (junction 100) : {i=i-1}
  (junction 73) -> (junction 79) [order 3] : {x=arrX[0]}
  (junction 100) -> (junction 104) [order 3] : {x=arrX[0]}
  (junction 79) -> (junction 90)
  (junction 104) -> (junction 110)
  (junction 73) -> (junction 75) [order 1] : [y>=arrY[i]]
      | {x=arrX[i]+(y-arrY[i])*(arrX[i+1]-arrX[i])/(arrY[i+1]-arrY[i])}
  (junction 100) -> (junction 107) [order 1] : [y<=arrY[i]]
      | {x=arrX[i]+(y-arrY[i])*(arrX[i+1]-arrX[i])/(arrY[i+1]-arrY[i])}
  (junction 75) -> (junction 90)
  (junction 107) -> (junction 110)
  (junction 90) -> (junction 113)
  (junction 110) -> (junction 112)
  (junction 113) -> (junction 112)
  (junction 112) -> (junction 118) : {err=1}
  data: arrX input; arrY input; i local uint8; len local uint8; xInc local uint8; yInc local uint8; y input; x output; err output
